simulink model "TimeConstantID"  (R2020a)
settings: Solver=VariableStepAuto  StartTime=0.0  StopTime=10.0  RelTol=1e-3
settings Model: Creator=Acer  LastModifiedBy=Acer

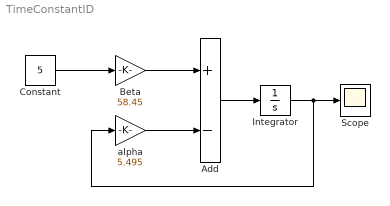
== system TimeConstantID ==
  Add : Sum  Inputs=+-
  Beta : Gain  Gain=58.45
  Constant : Constant  Value=5
  Integrator : Integrator
  Scope : Scope
  alpha : Gain  Gain=5.495
  wires:
  Constant/1 -> Beta/1
  Beta/1 -> Add/1
  alpha/1 -> Add/2
  Add/1 -> Integrator/1
  Integrator/1 -> alpha/1, Scope/1
